simulink model "sampleModel342"  (R2021b)
settings: Solver=VariableStepAuto  StartTime=0.0  StopTime=10.0  RelTol=1e-3
undefined symbols (not defined in the file or in its folder): DiscIntNeverNeededParam, magnitude
libraries: simulink x4
settings Model: Creator=user  LastModifiedBy=user

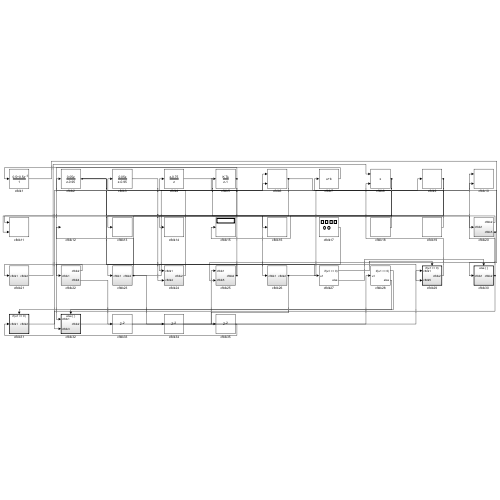
[thumbnail: Simulink's stored preview of the top-level diagram]
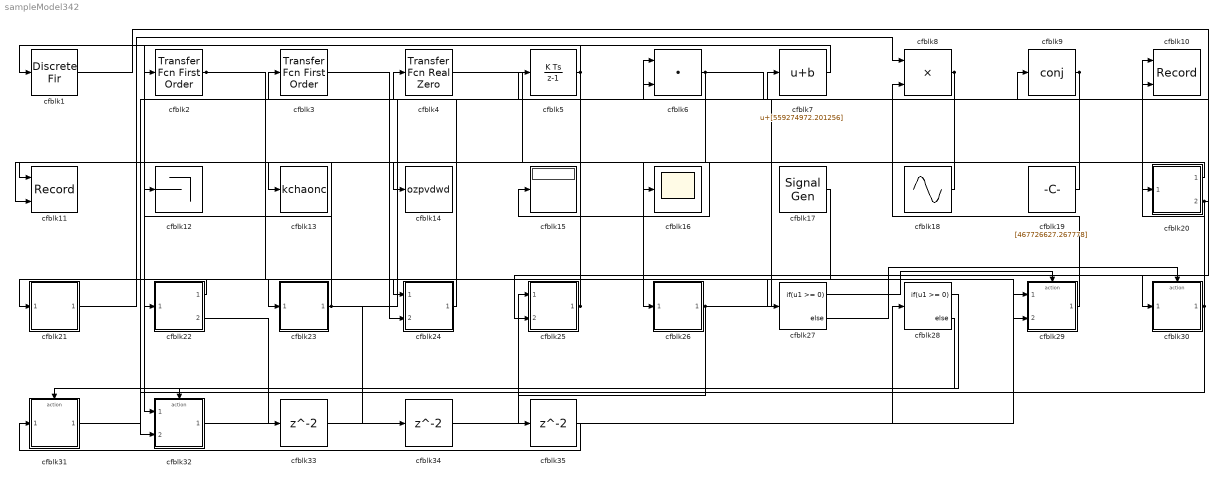
== system sampleModel342 ==
  cfblk1 : DiscreteFir  SampleTime=1
  cfblk10 : Record  FileSettingsInternal="{\"entries\":[{\"content\":{\"excelSettings\":{\"content\":{},\"type\":\"Streamout.ExcelSettings\"}},\"type\":\"Streamout.FileSettingStorage\",\"uuid\":\"248e99ca-0bf1-43f8-a27f-3f0ab8289ceb\"}],\"packageUris\":[\"http://schema.mathworks.com/mf0/streamout_blocks/R2020a\"],\"version\":\"1.0\"}"  Layout=[1 1]  SignalsInternal="{\"entries\":[{\"content\":{\"signals\":[{\"content\":{\"blockPath\":[\"sampleModel342/cfblk10\"],\"channel\":[],\"dimensions\":[1],\"domain\":\"sampleModel342/cfblk10\",\"lineColor\":\"#a2142f\",\"plots\":[1],\"port\":1,\"sid\":[\"\"],\"signalID\":14421,\"signalName\":\"cfblk30\"},\"type\":\"RecordBlkView.Signal\",\"uuid\":\"d9b59135-251b-4bec-994f-0fa0fefb7e07\"},{\"content\":{\"blockPath\":[\"sampleModel342/cfblk10\"],\"channel\":[],\"dimensions\":[1],\"domain\":\"sampleModel342/cfblk10\",\"lineColor\":\"#139fff\",\"plots\":[1],\"port\":2,\"sid\":[\"\"],\"signalID\":14425,\"signalName\":\"cfblk6\"},\"type\":\"RecordBlkView.Signal\",\"uuid\":\"8d29d2f0-21bc-4436-93a2-3ccd25c879c9\"}]},\"type\":\"RecordBlkView.InputSignals\",\"uuid\":\"ab0ed54c-9cdc-4317-96df-334b016bda0d\"}],\"packageUris\":[\"http://schema.mathworks.com/mf0/streamout_blocks/R2020a\"],\"version\":\"1.0\"}"  VisualizationBindings="{\"xyplotplugin\":{\"info\":[{\"series\":[{\"bindingParametersList\":[{\"parameter\":\"X-Axis\",\"signalID\":14421,\"signalName\":\"cfblk30\"},{\"parameter\":\"Y-Axis\",\"signalID\":14425,\"signalName\":\"cfblk6\"}],\"seriesID\":36592}],\"subplotID\":1}]}}"  CompatibilityTag=XY
  cfblk11 : Record  FileSettingsInternal="{\"entries\":[{\"content\":{\"excelSettings\":{\"content\":{},\"type\":\"Streamout.ExcelSettings\"}},\"type\":\"Streamout.FileSettingStorage\",\"uuid\":\"19ef1b9e-6b33-46a3-9c50-434e4abbd69f\"}],\"packageUris\":[\"http://schema.mathworks.com/mf0/streamout_blocks/R2020a\"],\"version\":\"1.0\"}"  Layout=[1 1]  SignalsInternal="{\"entries\":[{\"content\":{\"signals\":[{\"content\":{\"blockPath\":[\"sampleModel342/cfblk11\"],\"channel\":[],\"dimensions\":[1],\"domain\":\"sampleModel342/cfblk11\",\"lineColor\":\"#a2142f\",\"plots\":[1],\"port\":1,\"sid\":[\"\"],\"signalID\":14429,\"signalName\":\"cfblk8\"},\"type\":\"RecordBlkView.Signal\",\"uuid\":\"be962952-ad96-4c92-b5d7-7e2e660a1229\"},{\"content\":{\"blockPath\":[\"sampleModel342/cfblk11\"],\"channel\":[],\"dimensions\":[1],\"domain\":\"sampleModel342/cfblk11\",\"lineColor\":\"#139fff\",\"plots\":[1],\"port\":2,\"sid\":[\"\"],\"signalID\":14433,\"signalName\":\"cfblk5\"},\"type\":\"RecordBlkView.Signal\",\"uuid\":\"ae99e458-aec8-4f2c-bd18-5f78f3f2a416\"}]},\"type\":\"RecordBlkView.InputSignals\",\"uuid\":\"fe280051-e1d6-4a47-981a-40af06ef27c7\"}],\"packageUris\":[\"http://schema.mathworks.com/mf0/streamout_blocks/R2020a\"],\"version\":\"1.0\"}"  VisualizationBindings="{\"xyplotplugin\":{\"info\":[{\"series\":[{\"bindingParametersList\":[{\"parameter\":\"X-Axis\",\"signalID\":14429,\"signalName\":\"cfblk8\"},{\"parameter\":\"Y-Axis\",\"signalID\":14433,\"signalName\":\"cfblk5\"}],\"seriesID\":46883}],\"subplotID\":1}]}}"  CompatibilityTag=XY
  cfblk12 : Terminator
  cfblk13 : ToWorkspace  VariableName=kchaonc  SaveFormat=Timeseries  SampleTime=-1
  cfblk14 : ToWorkspace  VariableName=ozpvdwd  SaveFormat=Timeseries  SampleTime=-1
  cfblk15 : Display
  cfblk16 : Scope
  cfblk17 : SignalGenerator  WaveForm=square  Amplitude=[-928603519.193990]
  cfblk18 : Sin  Amplitude=[881557593.606640]  Bias=[-640828172.806162]  SampleTime=0
  cfblk19 : Constant  Value=[467726627.267778]  SampleTime=1
  cfblk2 : simulink/Discrete/Transfer Fcn First Order  PoleZ=0.95  ICPrevOutput=0.0  DoSatur=off
  cfblk20 : Subsystem
  cfblk21 : Subsystem
  cfblk22 : Subsystem
  cfblk23 : Subsystem
  cfblk24 : Subsystem
  cfblk25 : Subsystem
  cfblk26 : Subsystem
  cfblk27 : If  IfExpression=u1 >= 0  SampleTime=1
  cfblk28 : If  IfExpression=u1 >= 0  SampleTime=1
  cfblk29 : Subsystem  TreatAsAtomicUnit=on
  cfblk3 : simulink/Discrete/Transfer Fcn First Order  PoleZ=0.95  ICPrevOutput=0.0  DoSatur=off
  cfblk30 : Subsystem  TreatAsAtomicUnit=on
  cfblk31 : Subsystem  TreatAsAtomicUnit=on
  cfblk32 : Subsystem  TreatAsAtomicUnit=on
  cfblk33 : Delay  SampleTime=1
  cfblk34 : Delay  SampleTime=1
  cfblk35 : Delay  SampleTime=1
  cfblk4 : simulink/Discrete/Transfer Fcn Real Zero  ZeroZ=0.75  ICPrevInput=0.0  DoSatur=off
      settings: SourceProductBaseCode=SL
  cfblk5 : DiscreteIntegrator  ICPrevOutput=DiscIntNeverNeededParam  ICPrevScaledInput=DiscIntNeverNeededParam
  cfblk6 : DotProduct  InputSameDT=on  OutDataTypeStr=Inherit: Inherit via internal rule
  cfblk7 : Bias  Bias=[559274972.201256]
  cfblk8 : Product  Inputs=**
  cfblk9 : Math  Operator=conj  SaturateOnIntegerOverflow=on
  wires:
  cfblk23/1(cfblk2) -> cfblk6/1, cfblk12/1, cfblk34/1
  cfblk5/1 -> cfblk32/1(cfblk1), cfblk11/2
  cfblk17/1 -> cfblk24/1(cfblk1)
  cfblk6/1 -> cfblk13/1, cfblk10/2
  cfblk21/1(cfblk2) -> cfblk8/1
  cfblk20/1(cfblk2) -> cfblk15/1
  cfblk4/1 -> cfblk26/1(cfblk1)
  cfblk29/1(cfblk2) -> cfblk8/2
  cfblk3/1 -> cfblk24/2(cfblk4)
  cfblk1/1 -> cfblk30/1(cfblk1)
  cfblk24/1(cfblk2) -> cfblk2/1
  cfblk30/1(cfblk2) -> cfblk10/1, cfblk32/2(cfblk3)
  cfblk26/1(cfblk2) -> cfblk9/1, cfblk35/1
  cfblk31/1(cfblk2) -> cfblk6/2
  cfblk18/1 -> cfblk3/1
  cfblk7/1 -> cfblk1/1
  cfblk25/1(cfblk2) -> cfblk22/1(cfblk1), cfblk4/1
  cfblk2/1 -> cfblk20/1(cfblk1), cfblk27/1, cfblk29/2(cfblk5)
  cfblk9/1 -> cfblk23/1(cfblk1), cfblk14/1
  cfblk20/2(cfblk5) -> cfblk5/1, cfblk25/2(cfblk5)
  cfblk32/1(cfblk2) -> cfblk25/1(cfblk1)
  cfblk19/1 -> cfblk7/1
  cfblk8/1 -> cfblk16/1, cfblk11/1
  cfblk22/1(cfblk2) -> cfblk21/1(cfblk1)
  cfblk27/1 -> cfblk29/Action
  cfblk27/2 -> cfblk30/Action
  cfblk28/1 -> cfblk31/Action
  cfblk28/2 -> cfblk32/Action
  cfblk22/2(cfblk4) -> cfblk33/1
  cfblk33/1 -> cfblk28/1
  cfblk34/1 -> cfblk29/1(cfblk1)
  cfblk35/1 -> cfblk31/1(cfblk1)

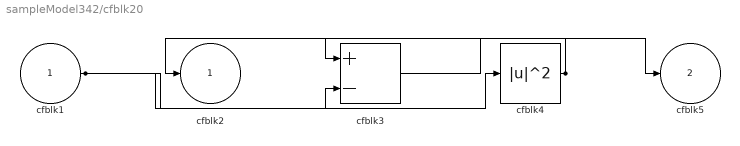
== system sampleModel342/cfblk20 ==
  cfblk1 : Inport
  cfblk3 : Sum  Inputs=+-
  cfblk4 : Math  Operator=magnitude^2  SaturateOnIntegerOverflow=on
  cfblk2 : Outport
  cfblk5 : Outport  Port=2
  wires:
  cfblk4/1 -> cfblk2/1, cfblk3/1
  cfblk1/1 -> cfblk4/1, cfblk3/2
  cfblk3/1 -> cfblk5/1

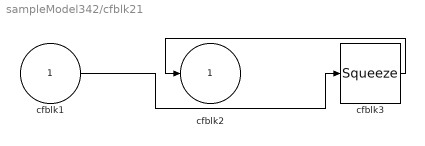
== system sampleModel342/cfblk21 ==
  cfblk1 : Inport
  cfblk3 : Squeeze
  cfblk2 : Outport
  wires:
  cfblk3/1 -> cfblk2/1
  cfblk1/1 -> cfblk3/1

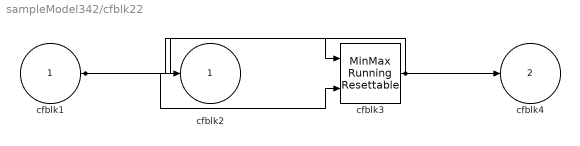
== system sampleModel342/cfblk22 ==
  cfblk1 : Inport
  cfblk3 : simulink/Math Operations/MinMax Running Resettable  Function=min  vinit=0.0
  cfblk2 : Outport
  cfblk4 : Outport  Port=2
  wires:
  cfblk3/1 -> cfblk4/1, cfblk2/1
  cfblk1/1 -> cfblk3/1, cfblk3/2

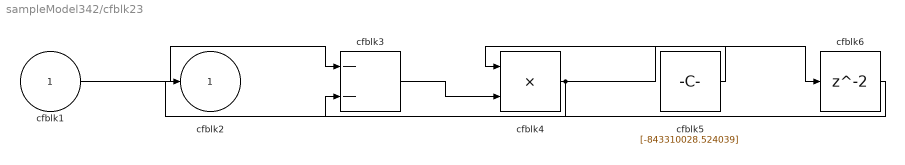
== system sampleModel342/cfblk23 ==
  cfblk1 : Inport
  cfblk3 : Sum  Inputs=--
  cfblk4 : Product
  cfblk5 : Constant  Value=[-843310028.524039]  SampleTime=1
  cfblk6 : Delay  SampleTime=1
  cfblk2 : Outport
  wires:
  cfblk5/1 -> cfblk4/1
  cfblk1/1 -> cfblk3/1
  cfblk4/1 -> cfblk2/1, cfblk6/1
  cfblk3/1 -> cfblk4/2
  cfblk6/1 -> cfblk3/2

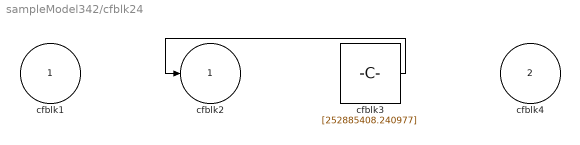
== system sampleModel342/cfblk24 ==
  cfblk1 : Inport
  cfblk4 : Inport  Port=2
  cfblk3 : Constant  Value=[252885408.240977]  SampleTime=1
  cfblk2 : Outport
  wires:
  cfblk3/1 -> cfblk2/1

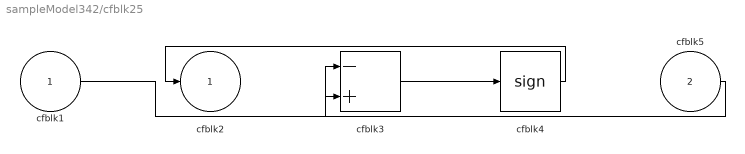
== system sampleModel342/cfblk25 ==
  cfblk1 : Inport
  cfblk5 : Inport  Port=2
  cfblk3 : Sum  Inputs=-+
  cfblk4 : Signum
  cfblk2 : Outport
  wires:
  cfblk3/1 -> cfblk4/1
  cfblk4/1 -> cfblk2/1
  cfblk1/1 -> cfblk3/1
  cfblk5/1 -> cfblk3/2

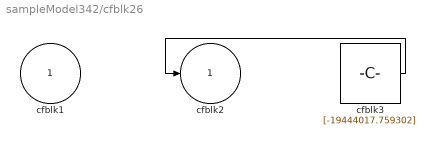
== system sampleModel342/cfblk26 ==
  cfblk1 : Inport
  cfblk3 : Constant  Value=[-19444017.759302]  SampleTime=1
  cfblk2 : Outport
  wires:
  cfblk3/1 -> cfblk2/1

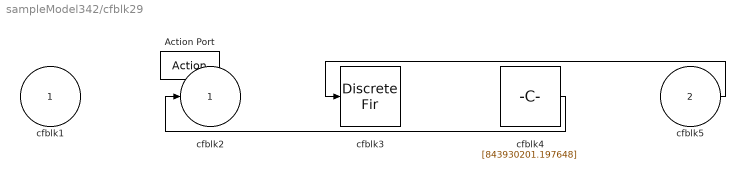
== system sampleModel342/cfblk29 ==
  cfblk1 : Inport
  cfblk5 : Inport  Port=2
  Action Port : ActionPort  ActionPortLabel=if(u1 >= 0)
  cfblk3 : DiscreteFir
  cfblk4 : Constant  Value=[843930201.197648]  SampleTime=1
  cfblk2 : Outport
  wires:
  cfblk5/1 -> cfblk3/1
  cfblk4/1 -> cfblk2/1

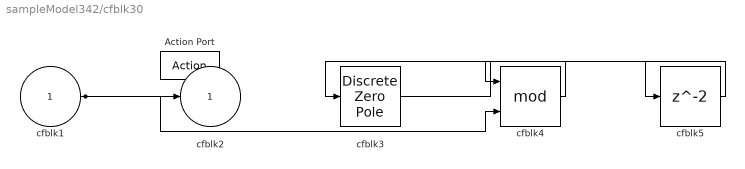
== system sampleModel342/cfblk30 ==
  cfblk1 : Inport
  Action Port : ActionPort  ActionPortLabel=else
  cfblk3 : DiscreteZeroPole  Poles=[0 0.5]  Gain=1  SampleTime=-1
  cfblk4 : Math  Operator=mod  SaturateOnIntegerOverflow=on
  cfblk5 : Delay
  cfblk2 : Outport
  wires:
  cfblk4/1 -> cfblk3/1
  cfblk1/1 -> cfblk2/1, cfblk4/2
  cfblk3/1 -> cfblk5/1
  cfblk5/1 -> cfblk4/1

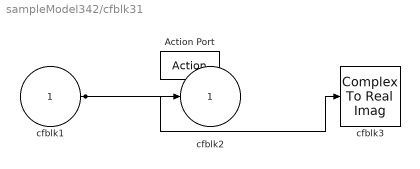
== system sampleModel342/cfblk31 ==
  cfblk1 : Inport
  Action Port : ActionPort  ActionPortLabel=if(u1 >= 0)
  cfblk3 : ComplexToRealImag
  cfblk2 : Outport
  wires:
  cfblk1/1 -> cfblk2/1, cfblk3/1

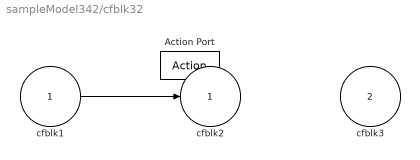
== system sampleModel342/cfblk32 ==
  cfblk1 : Inport
  cfblk3 : Inport  Port=2
  Action Port : ActionPort  ActionPortLabel=else
  cfblk2 : Outport
  wires:
  cfblk1/1 -> cfblk2/1
